simulink model "g2simulink"  (R2023b)
settings: Solver=FixedStepAuto  StartTime=0.0  StopTime=450  FixedStep=1e-5  RelTol=1e-3
values from neighbouring files (symbols this model uses):
  C2A = [(1.5215+0.380/s), (-0.291-0.0727/s), (0.0052+0.0013/s) ... (first row only)    [g2.m]
  C2B = [(1.23+0.183/s), (-0.0716-0.0220/s), (0.0017+(2.08*10^(-4))/s) ... (first row only)    [g2.m]
  C2C = [(1.31+0.354/s), (-0.0135-0.0582/s), (0.0207+0.0026/s) ... (first row only)    [g2.m]
  G2 = [0.66/(6.7*s+1), -0.61/(8.64*s+1), -0.0049/(9.06*s+1) ... (first row only)    [g2.m]
libraries: cstblocks x54
settings Model: Creator=klysm  LastModifiedBy=klysm

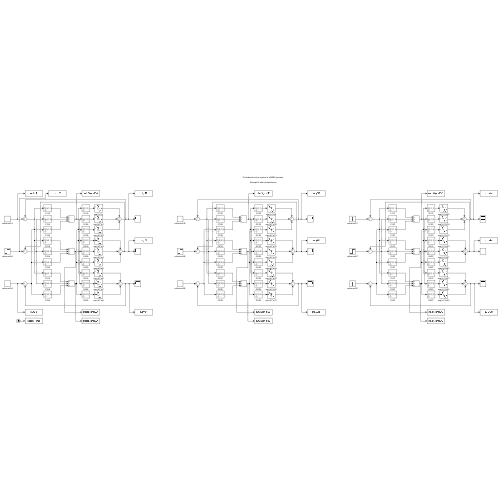
[thumbnail: Simulink's stored preview of the top-level diagram]
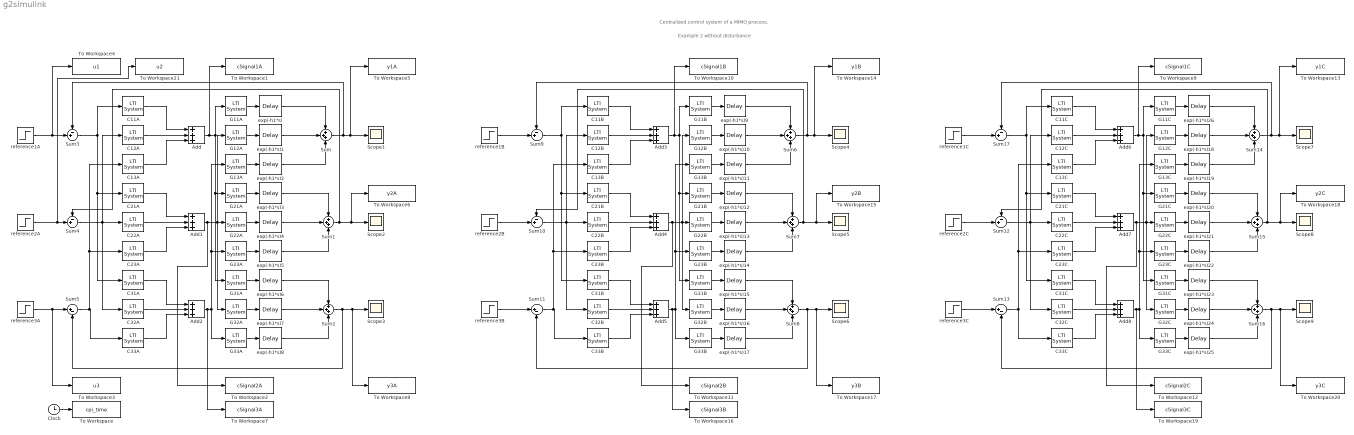
== system g2simulink ==
  note: Example 2 without disturbance
  note: Centralized control system of a MIMO process.
  Add{,1..8} (9 alike) : Sum  Inputs=+++
  C11A : cstblocks/LTI System  sys=C2A(1,1)  IC=[]  PadeOrder=0
  C11B : cstblocks/LTI System  sys=C2B(1,1)  IC=[]  PadeOrder=0
  C11C : cstblocks/LTI System  sys=C2C(1,1)  IC=[]  PadeOrder=0
  C12A : cstblocks/LTI System  sys=C2A(1,2)  IC=[]  PadeOrder=0
  C12B : cstblocks/LTI System  sys=C2B(1,2)  IC=[]  PadeOrder=0
  C12C : cstblocks/LTI System  sys=C2C(1,2)  IC=[]  PadeOrder=0
  C13A : cstblocks/LTI System  sys=C2A(1,3)  IC=[]  PadeOrder=0
  C13B : cstblocks/LTI System  sys=C2B(1,3)  IC=[]  PadeOrder=0
  C13C : cstblocks/LTI System  sys=C2C(1,3)  IC=[]  PadeOrder=0
  C21A : cstblocks/LTI System  sys=C2A(2,1)  IC=[]  PadeOrder=0
  C21B : cstblocks/LTI System  sys=C2B(2,1)  IC=[]  PadeOrder=0
  C21C : cstblocks/LTI System  sys=C2C(2,1)  IC=[]  PadeOrder=0
  C22A : cstblocks/LTI System  sys=C2A(2,2)  IC=[]  PadeOrder=0
  C22B : cstblocks/LTI System  sys=C2B(2,2)  IC=[]  PadeOrder=0
  C22C : cstblocks/LTI System  sys=C2C(2,2)  IC=[]  PadeOrder=0
  C23A : cstblocks/LTI System  sys=C2A(2,3)  IC=[]  PadeOrder=0
  C23B : cstblocks/LTI System  sys=C2B(2,3)  IC=[]  PadeOrder=0
  C23C : cstblocks/LTI System  sys=C2C(2,3)  IC=[]  PadeOrder=0
  C31A : cstblocks/LTI System  sys=C2A(3,1)  IC=[]  PadeOrder=0
  C31B : cstblocks/LTI System  sys=C2B(3,1)  IC=[]  PadeOrder=0
  C31C : cstblocks/LTI System  sys=C2C(3,1)  IC=[]  PadeOrder=0
  C32A : cstblocks/LTI System  sys=C2A(3,2)  IC=[]  PadeOrder=0
  C32B : cstblocks/LTI System  sys=C2B(3,2)  IC=[]  PadeOrder=0
  C32C : cstblocks/LTI System  sys=C2C(3,2)  IC=[]  PadeOrder=0
  C33A : cstblocks/LTI System  sys=C2A(3,3)  IC=[]  PadeOrder=0
  C33B : cstblocks/LTI System  sys=C2B(3,3)  IC=[]  PadeOrder=0
  C33C : cstblocks/LTI System  sys=C2C(3,3)  IC=[]  PadeOrder=0
  Clock : Clock
  G11A : cstblocks/LTI System  sys=G2(1,1)  IC=[]  PadeOrder=0
  G11B : cstblocks/LTI System  sys=G2(1,1)  IC=[]  PadeOrder=0
  G11C : cstblocks/LTI System  sys=G2(1,1)  IC=[]  PadeOrder=0
  G12A : cstblocks/LTI System  sys=G2(1,2)  IC=[]  PadeOrder=0
  G12B : cstblocks/LTI System  sys=G2(1,2)  IC=[]  PadeOrder=0
  G12C : cstblocks/LTI System  sys=G2(1,2)  IC=[]  PadeOrder=0
  G13A : cstblocks/LTI System  sys=G2(1,3)  IC=[]  PadeOrder=0
  G13B : cstblocks/LTI System  sys=G2(1,3)  IC=[]  PadeOrder=0
  G13C : cstblocks/LTI System  sys=G2(1,3)  IC=[]  PadeOrder=0
  G21A : cstblocks/LTI System  sys=G2(2,1)  IC=[]  PadeOrder=0
  G21B : cstblocks/LTI System  sys=G2(2,1)  IC=[]  PadeOrder=0
  G21C : cstblocks/LTI System  sys=G2(2,1)  IC=[]  PadeOrder=0
  G22A : cstblocks/LTI System  sys=G2(2,2)  IC=[]  PadeOrder=0
  G22B : cstblocks/LTI System  sys=G2(2,2)  IC=[]  PadeOrder=0
  G22C : cstblocks/LTI System  sys=G2(2,2)  IC=[]  PadeOrder=0
  G23A : cstblocks/LTI System  sys=G2(2,3)  IC=[]  PadeOrder=0
  G23B : cstblocks/LTI System  sys=G2(2,3)  IC=[]  PadeOrder=0
  G23C : cstblocks/LTI System  sys=G2(2,3)  IC=[]  PadeOrder=0
  G31A : cstblocks/LTI System  sys=G2(3,1)  IC=[]  PadeOrder=0
  G31B : cstblocks/LTI System  sys=G2(3,1)  IC=[]  PadeOrder=0
  G31C : cstblocks/LTI System  sys=G2(3,1)  IC=[]  PadeOrder=0
  G32A : cstblocks/LTI System  sys=G2(3,2)  IC=[]  PadeOrder=0
  G32B : cstblocks/LTI System  sys=G2(3,2)  IC=[]  PadeOrder=0
  G32C : cstblocks/LTI System  sys=G2(3,2)  IC=[]  PadeOrder=0
  G33A : cstblocks/LTI System  sys=G2(3,3)  IC=[]  PadeOrder=0
  G33B : cstblocks/LTI System  sys=G2(3,3)  IC=[]  PadeOrder=0
  G33C : cstblocks/LTI System  sys=G2(3,3)  IC=[]  PadeOrder=0
  Scope{1..9} (9 alike) : Scope
  Sum{,1..2,6..8,14..16} (9 alike) : Sum  Inputs=+++
  Sum{3..4,9..10,12,17} (6 alike) : Sum  Inputs=-+|
  Sum11 : Sum  Inputs=|+-
  Sum13 : Sum  Inputs=|+-
  Sum5 : Sum  Inputs=|+-
  To Workspace : ToWorkspace  VariableName=cpi_time  SampleTime=-1
  To Workspace1 : ToWorkspace  VariableName=cSignal1A  SampleTime=-1
  To Workspace10 : ToWorkspace  VariableName=cSignal1B  SampleTime=-1
  To Workspace11 : ToWorkspace  VariableName=cSignal2B  SampleTime=-1
  To Workspace12 : ToWorkspace  VariableName=cSignal2C  SampleTime=-1
  To Workspace13 : ToWorkspace  VariableName=y1C  SampleTime=-1
  To Workspace14 : ToWorkspace  VariableName=y1B  SampleTime=-1
  To Workspace15 : ToWorkspace  VariableName=y2B  SampleTime=-1
  To Workspace16 : ToWorkspace  VariableName=cSignal3B  SampleTime=-1
  To Workspace17 : ToWorkspace  VariableName=y3B  SampleTime=-1
  To Workspace18 : ToWorkspace  VariableName=y2C  SampleTime=-1
  To Workspace19 : ToWorkspace  VariableName=cSignal3C  SampleTime=-1
  To Workspace2 : ToWorkspace  VariableName=cSignal2A  SampleTime=-1
  To Workspace20 : ToWorkspace  VariableName=y3C  SampleTime=-1
  To Workspace21 : ToWorkspace  VariableName=u2  SampleTime=-1
  To Workspace3 : ToWorkspace  VariableName=u3  SampleTime=-1
  To Workspace4 : ToWorkspace  VariableName=u1  SampleTime=-1
  To Workspace5 : ToWorkspace  VariableName=y1A  SampleTime=-1
  To Workspace6 : ToWorkspace  VariableName=y2A  SampleTime=-1
  To Workspace7 : ToWorkspace  VariableName=cSignal3A  SampleTime=-1
  To Workspace8 : ToWorkspace  VariableName=y3A  SampleTime=-1
  To Workspace9 : ToWorkspace  VariableName=cSignal1C  SampleTime=-1
  exp(-h1*s) : TransportDelay  DelayTime=2.6
  exp(-h1*s)1 : TransportDelay  DelayTime=3.5
  exp(-h1*s)10 : TransportDelay  DelayTime=3.5
  exp(-h1*s){2,8,11,17,19,25} (6 alike) : TransportDelay
  exp(-h1*s)12 : TransportDelay  DelayTime=6.5
  exp(-h1*s)13 : TransportDelay  DelayTime=3
  exp(-h1*s)14 : TransportDelay  DelayTime=1.2
  exp(-h1*s){6..7,15..16,23..24} (6 alike) : TransportDelay  DelayTime=7
  exp(-h1*s)18 : TransportDelay  DelayTime=3.5
  exp(-h1*s)20 : TransportDelay  DelayTime=6.5
  exp(-h1*s)21 : TransportDelay  DelayTime=3
  exp(-h1*s)22 : TransportDelay  DelayTime=1.2
  exp(-h1*s)26 : TransportDelay  DelayTime=2.6
  exp(-h1*s)3 : TransportDelay  DelayTime=6.5
  exp(-h1*s)4 : TransportDelay  DelayTime=3
  exp(-h1*s)5 : TransportDelay  DelayTime=1.2
  exp(-h1*s)9 : TransportDelay  DelayTime=2.6
  reference1A : Step  Time=0  SampleTime=0
  reference1B : Step  Time=0  SampleTime=0
  reference1C : Step  Time=0  SampleTime=0
  reference2A : Step  Time=150  SampleTime=0
  reference2B : Step  Time=150  SampleTime=0
  reference2C : Step  Time=150  SampleTime=0
  reference3A : Step  Time=300  SampleTime=0
  reference3B : Step  Time=300  SampleTime=0
  reference3C : Step  Time=300  SampleTime=0
  wires:
  G21A/1 -> exp(-h1*s)3/1
  G13A/1 -> exp(-h1*s)2/1
  G12A/1 -> exp(-h1*s)1/1
  G11A/1 -> exp(-h1*s)/1
  G33A/1 -> exp(-h1*s)8/1
  G32A/1 -> exp(-h1*s)7/1
  G31A/1 -> exp(-h1*s)6/1
  G23A/1 -> exp(-h1*s)5/1
  G22A/1 -> exp(-h1*s)4/1
  exp(-h1*s)8/1 -> Sum2/3
  exp(-h1*s)7/1 -> Sum2/2
  exp(-h1*s)6/1 -> Sum2/1
  exp(-h1*s)5/1 -> Sum1/3
  exp(-h1*s)4/1 -> Sum1/2
  exp(-h1*s)3/1 -> Sum1/1
  exp(-h1*s)2/1 -> Sum/3
  exp(-h1*s)1/1 -> Sum/2
  exp(-h1*s)/1 -> Sum/1
  Add/1 -> To Workspace1/1, G31A/1, G21A/1, G11A/1
  Add1/1 -> To Workspace2/1, G32A/1, G22A/1, G12A/1
  Add2/1 -> To Workspace7/1, G13A/1, G23A/1, G33A/1
  C11A/1 -> Add/1
  C12A/1 -> Add/2
  C13A/1 -> Add/3
  C22A/1 -> Add1/2
  C21A/1 -> Add1/1
  C23A/1 -> Add1/3
  C31A/1 -> Add2/1
  C32A/1 -> Add2/2
  C33A/1 -> Add2/3
  Sum3/1 -> C11A/1, C31A/1, C21A/1
  reference1A/1 -> To Workspace4/1, Sum3/2
  reference2A/1 -> To Workspace21/1, Sum4/2
  reference3A/1 -> Sum5/1, To Workspace3/1
  Sum4/1 -> C32A/1, C12A/1, C22A/1
  Sum5/1 -> C13A/1, C23A/1, C33A/1
  Sum/1 -> Sum3/1, Scope1/1, To Workspace5/1
  Sum1/1 -> Sum4/1, To Workspace6/1, Scope2/1
  Sum2/1 -> Sum5/2, To Workspace8/1, Scope3/1
  Clock/1 -> To Workspace/1
  Sum8/1 -> Sum11/2, To Workspace17/1, Scope6/1
  exp(-h1*s)11/1 -> Sum6/3
  Sum10/1 -> C32B/1, C12B/1, C22B/1
  Sum11/1 -> C13B/1, C23B/1, C33B/1
  exp(-h1*s)16/1 -> Sum8/2
  Sum7/1 -> Sum10/1, To Workspace15/1, Scope5/1
  C23B/1 -> Add4/3
  G23B/1 -> exp(-h1*s)14/1
  exp(-h1*s)12/1 -> Sum7/1
  exp(-h1*s)10/1 -> Sum6/2
  reference3B/1 -> Sum11/1
  C21B/1 -> Add4/1
  exp(-h1*s)15/1 -> Sum8/1
  reference2B/1 -> Sum10/2
  Sum9/1 -> C11B/1, C31B/1, C21B/1
  G11B/1 -> exp(-h1*s)9/1
  G22B/1 -> exp(-h1*s)13/1
  reference1B/1 -> Sum9/2
  C22B/1 -> Add4/2
  Add5/1 -> To Workspace16/1, G13B/1, G23B/1, G33B/1
  C11B/1 -> Add3/1
  Add3/1 -> To Workspace10/1, G31B/1, G21B/1, G11B/1
  C31B/1 -> Add5/1
  C33B/1 -> Add5/3
  G33B/1 -> exp(-h1*s)17/1
  exp(-h1*s)9/1 -> Sum6/1
  C13B/1 -> Add3/3
  C32B/1 -> Add5/2
  Add4/1 -> To Workspace11/1, G32B/1, G22B/1, G12B/1
  C12B/1 -> Add3/2
  G31B/1 -> exp(-h1*s)15/1
  exp(-h1*s)14/1 -> Sum7/3
  exp(-h1*s)13/1 -> Sum7/2
  Sum6/1 -> Sum9/1, Scope4/1, To Workspace14/1
  G12B/1 -> exp(-h1*s)10/1
  exp(-h1*s)17/1 -> Sum8/3
  G32B/1 -> exp(-h1*s)16/1
  G21B/1 -> exp(-h1*s)12/1
  G13B/1 -> exp(-h1*s)11/1
  exp(-h1*s)21/1 -> Sum15/2
  G32C/1 -> exp(-h1*s)24/1
  exp(-h1*s)25/1 -> Sum16/3
  G21C/1 -> exp(-h1*s)20/1
  Sum14/1 -> Sum17/1, Scope7/1, To Workspace13/1
  G12C/1 -> exp(-h1*s)18/1
  C31C/1 -> Add8/1
  C13C/1 -> Add6/3
  G31C/1 -> exp(-h1*s)23/1
  exp(-h1*s)26/1 -> Sum14/1
  C12C/1 -> Add6/2
  Add7/1 -> To Workspace12/1, G32C/1, G22C/1, G12C/1
  C33C/1 -> Add8/3
  C32C/1 -> Add8/2
  G33C/1 -> exp(-h1*s)25/1
  C11C/1 -> Add6/1
  reference1C/1 -> Sum17/2
  Add8/1 -> To Workspace19/1, G13C/1, G23C/1, G33C/1
  G22C/1 -> exp(-h1*s)21/1
  Sum17/1 -> C11C/1, C31C/1, C21C/1
  reference3C/1 -> Sum13/1
  G11C/1 -> exp(-h1*s)26/1
  exp(-h1*s)18/1 -> Sum14/2
  G13C/1 -> exp(-h1*s)19/1
  exp(-h1*s)20/1 -> Sum15/1
  G23C/1 -> exp(-h1*s)22/1
  Sum12/1 -> C32C/1, C12C/1, C22C/1
  exp(-h1*s)23/1 -> Sum16/1
  Sum15/1 -> Sum12/1, To Workspace18/1, Scope8/1
  exp(-h1*s)24/1 -> Sum16/2
  exp(-h1*s)19/1 -> Sum14/3
  Sum16/1 -> Sum13/2, To Workspace20/1, Scope9/1
  C23C/1 -> Add7/3
  exp(-h1*s)22/1 -> Sum15/3
  reference2C/1 -> Sum12/2
  C21C/1 -> Add7/1
  C22C/1 -> Add7/2
  Sum13/1 -> C13C/1, C23C/1, C33C/1
  Add6/1 -> To Workspace9/1, G31C/1, G21C/1, G11C/1
